simulink model "FinalProject"  (R2024b)
settings: Solver=VariableStepAuto  StartTime=0.0  StopTime=50  RelTol=1e-3
undefined symbols (not defined in the file): designMultirateFIR
libraries: dspvision x6, dspmlti4 x3, dspstat3 x2, dspsnks4 x1, dspadpt3 x1
settings Model: Creator=pniko  LastModifiedBy=pniko

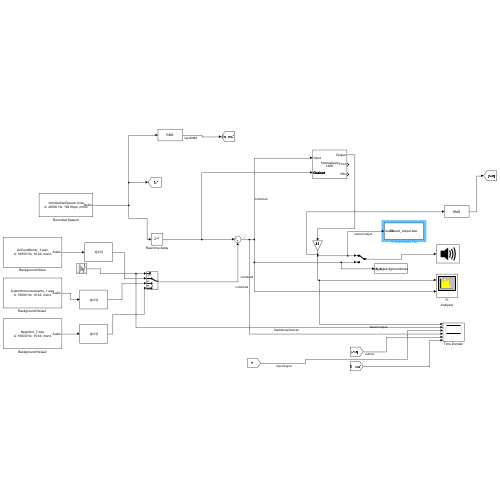
[thumbnail: Simulink's stored preview of the top-level diagram]
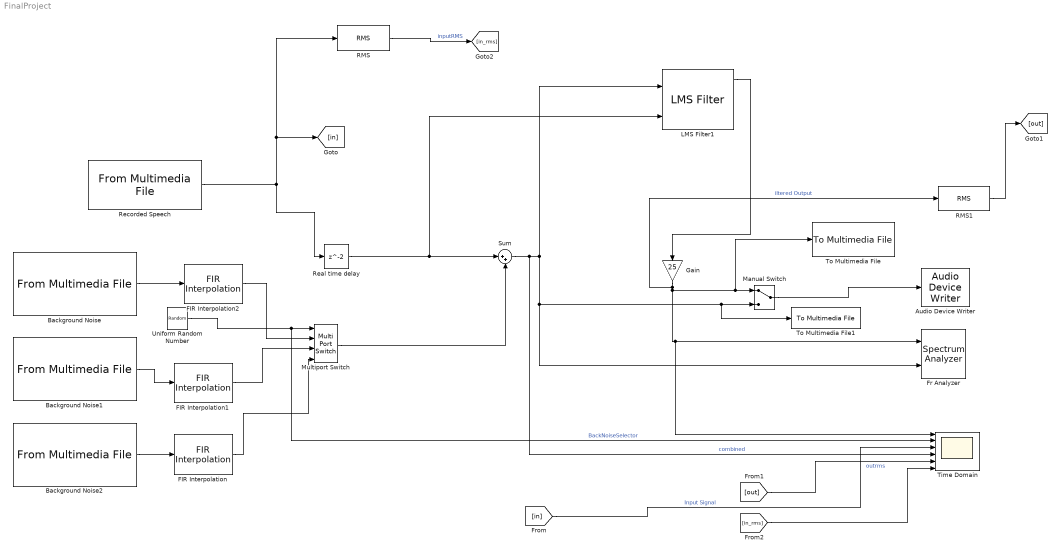
== system FinalProject ==
  Audio Device Writer : dspsnks4/Audio Device Writer  Driver=DirectSound  Device=Speakers (Realtek(R) Audio)  InheritSampleRate=on  SampleRate=48000  BitDepth=16-bit integer  BufferSize=4096  NumBuffers=10  DefaultOutputChannelMapping=on  OutputChannelMapping=1:2  OutputNumUnderrunSamples=off  DriverIdx=1  DeviceWarnFlag=''
  Background Noise : dspvision/From Multimedia File  inputFilename=C:\Users\pniko\OneDrive\Documents\NOISE\MS-SNSD-master\noise_test\AirConditioner_1.wav  readRange=[1 inf]  loop=on  numPlays=inf  outputStreams=Audio only  videoDataType=single  audioDataType=double  inheritSampleTime=on  userDefinedSampleTime=1/30  noAudioOutput=off  isIntensityVideo=off  fourcc=RGB  colorVideoFormat=Separate color signals  outputEOF=off  dataOrg=Column-major  audioFrameSize=16000  computeAudioFrameSize=off  outSamplingMode=Sample based
      settings: LibrarySourceBlock=audiosources/From Multimedia File
  Background Noise1 : dspvision/From Multimedia File  inputFilename=C:\Users\pniko\OneDrive\Documents\NOISE\MS-SNSD-master\noise_test\AirportAnnouncements_1.wav  readRange=[1 inf]  loop=on  numPlays=inf  outputStreams=Audio only  videoDataType=single  audioDataType=double  inheritSampleTime=on  userDefinedSampleTime=1/30  noAudioOutput=off  isIntensityVideo=off  fourcc=RGB  colorVideoFormat=Separate color signals  outputEOF=off  dataOrg=Column-major  audioFrameSize=16000  computeAudioFrameSize=off  outSamplingMode=Sample based
      settings: LibrarySourceBlock=audiosources/From Multimedia File
  Background Noise2 : dspvision/From Multimedia File  inputFilename=C:\Users\pniko\OneDrive\Documents\NOISE\MS-SNSD-master\noise_test\Neighbor_7.wav  readRange=[1 inf]  loop=on  numPlays=inf  outputStreams=Audio only  videoDataType=single  audioDataType=double  inheritSampleTime=on  userDefinedSampleTime=1/30  noAudioOutput=off  isIntensityVideo=off  fourcc=RGB  colorVideoFormat=Separate color signals  outputEOF=off  dataOrg=Column-major  audioFrameSize=16000  computeAudioFrameSize=off  outSamplingMode=Sample based
      settings: LibrarySourceBlock=audiosources/From Multimedia File
  FIR Interpolation : dspmlti4/FIR Interpolation  FilterSource=Auto  PrivateCoeffs=0  h=designMultirateFIR(3,1)  L=3  FilterObject=FINTERP  InputProcessing=Columns as channels (frame based)  framing=Enforce single-rate processing  outputBufInitCond=0  roundingMode=Floor  overflowMode=off  firstCoeffDataTypeStr=Inherit: Same word length as input  firstCoeffMin=[]  firstCoeffMax=[]  firstCoeffLastDataTypeStr=Inherit: Same word length as input  outputDataTypeStr=Inherit: Same as accumulator  outputMin=[]  outputMax=[]  outputLastDataTypeStr=Inherit: Same as accumulator
  FIR Interpolation1 : dspmlti4/FIR Interpolation  FilterSource=Auto  PrivateCoeffs=0  h=designMultirateFIR(3,1)  L=3  FilterObject=FINTERP  InputProcessing=Columns as channels (frame based)  framing=Enforce single-rate processing  outputBufInitCond=0  roundingMode=Floor  overflowMode=off  firstCoeffDataTypeStr=Inherit: Same word length as input  firstCoeffMin=[]  firstCoeffMax=[]  firstCoeffLastDataTypeStr=Inherit: Same word length as input  outputDataTypeStr=Inherit: Same as accumulator  outputMin=[]  outputMax=[]  outputLastDataTypeStr=Inherit: Same as accumulator
  FIR Interpolation2 : dspmlti4/FIR Interpolation  FilterSource=Auto  PrivateCoeffs=0  h=designMultirateFIR(3,1)  L=3  FilterObject=FINTERP  InputProcessing=Columns as channels (frame based)  framing=Enforce single-rate processing  outputBufInitCond=0  roundingMode=Floor  overflowMode=off  firstCoeffDataTypeStr=Inherit: Same word length as input  firstCoeffMin=[]  firstCoeffMax=[]  firstCoeffLastDataTypeStr=Inherit: Same word length as input  outputDataTypeStr=Inherit: Same as accumulator  outputMin=[]  outputMax=[]  outputLastDataTypeStr=Inherit: Same as accumulator
  Fr Analyzer : SpectrumAnalyzer  NumInputPorts=2  WindowPosition=[645.000000,50.000000,1197.000000,1000.000000,]  Visible=on  ScopeFrameLocation=window  ViewType=Spectrum and spectrogram  WindowInvariantSamplesPerUpdate=on  Span=48000  StartFrequency=-24000  StopFrequency=24000  YLimits=[-130.15043377,11.34598667]  ColorLimits=[-130.15043377,11.34598667]  ShowLegend=on  ExpandToolstrip=on
  Gain : Gain  Gain=25
  LMS Filter1 : dspadpt3/LMS Filter  Algo=Normalized LMS  L=150  stepflag=Dialog  mu=0.01  leakage=.001  ic=0  Adapt=off  resetflag=None  weights=on  addnparflag=off  roundingMode=Floor  overflowMode=off
  Manual Switch : ManualSwitch
  Multiport Switch : MultiPortSwitch  SaturateOnIntegerOverflow=off  InputSameDT=off
  RMS : dspstat3/RMS  run=off  directionMode=Each column  dimension=1  InputProcessing=Columns as channels (frame based)  reset_popup=None
  RMS1 : dspstat3/RMS  run=off  directionMode=Each column  dimension=1  InputProcessing=Columns as channels (frame based)  reset_popup=None
  Real time delay : Delay  InputProcessing=Columns as channels (frame based)
  Recorded Speech : dspvision/From Multimedia File  inputFilename=C:\Users\pniko\OneDrive\Documents\Sound Recordings\IntroductionSpeech.m4a  readRange=[1 inf]  loop=on  numPlays=5  outputStreams=Audio only  videoDataType=single  audioDataType=double  inheritSampleTime=on  userDefinedSampleTime=1/30  noAudioOutput=off  isIntensityVideo=off  fourcc=RGB  colorVideoFormat=Separate color signals  outputEOF=off  dataOrg=Column-major  audioFrameSize=48000  computeAudioFrameSize=off  outSamplingMode=Sample based
      settings: LibrarySourceBlock=audiosources/From Multimedia File
  Sum : Sum  Inputs=|++
  "Time Domain " : Scope  NumInputPorts=6
  To Multimedia File : dspvision/To Multimedia File  outputFilename=C:\Users\pniko\OneDrive\Documents\MATLAB\EGCP554\Source\filtered_output.wav  streamSelection=Audio only  videoCompressor=None (uncompressed)  audioCompressor=None (uncompressed)  imagePorts=One multidimensional signal  fileType=WAV  audioDatatype=16-bit integer  fourcc=RGB  audioBitRate=128  audioQuality=75  videoQuality=75  mj2000CompFactor=10
      settings: LibrarySourceBlock=dspsnks4/To Multimedia File
  To Multimedia File1 : dspvision/To Multimedia File  outputFilename=C:\Users\pniko\OneDrive\Documents\MATLAB\EGCP554\Source\Speech_w_backgroundnoise.wav  streamSelection=Audio only  videoCompressor=None (uncompressed)  audioCompressor=None (uncompressed)  imagePorts=One multidimensional signal  fileType=WAV  audioDatatype=16-bit integer  fourcc=RGB  audioBitRate=128  audioQuality=75  videoQuality=75  mj2000CompFactor=10
      settings: LibrarySourceBlock=dspsnks4/To Multimedia File
  Uniform Random Number : UniformRandomNumber  Minimum=1  Maximum=4  SampleTime=8
  wires:
  Recorded Speech/1 -> Real time delay/1, RMS/1, [in]
  Real time delay/1 -> LMS Filter1/2, Sum/1
  Sum/1 -> "Time Domain "/4, LMS Filter1/1, To Multimedia File1/1, Manual Switch/2, Fr Analyzer/2  "combined"
  Multiport Switch/1 -> Sum/2
  Background Noise/1 -> FIR Interpolation2/1
  FIR Interpolation2/1 -> Multiport Switch/2
  Background Noise1/1 -> FIR Interpolation1/1
  FIR Interpolation1/1 -> Multiport Switch/3
  Background Noise2/1 -> FIR Interpolation/1
  FIR Interpolation/1 -> Multiport Switch/4
  Uniform Random Number/1 -> "Time Domain "/2, Multiport Switch/1  "BackNoiseSelector"
  Gain/1 -> To Multimedia File/1, Manual Switch/1, "Time Domain "/1, Fr Analyzer/1, RMS1/1  "iltered Output"
  [in] -> "Time Domain "/3  "Input Signal"
  LMS Filter1/1 -> Gain/1
  RMS1/1 -> [out]
  RMS/1 -> [in_rms]  "inputRMS"
  [out] -> "Time Domain "/5  "outrms"
  [in_rms] -> "Time Domain "/6
  Manual Switch/1 -> Audio Device Writer/1
